simulink model "COMP_POS_CMD"  (R2026b)
settings: Solver=VariableStepAuto
libraries: simulink_extras x1
settings Model: Creator=bhorton  LastModifiedBy=bhorton

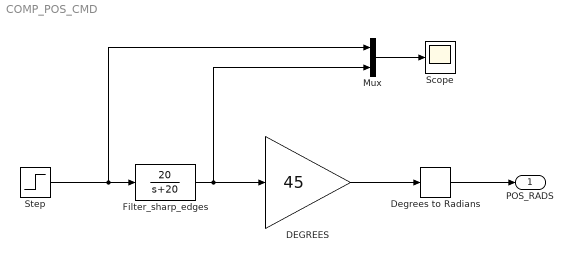
== system COMP_POS_CMD ==
  DEGREES : Gain  Gain=45
  Degrees to Radians : simulink_extras/Transformations/Degrees to Radians
  Filter_sharp_edges : TransferFcn  Numerator=[20]  Denominator=[1 20]
  Mux : Mux  Inputs=2
  Scope : Scope
      settings: ActiveDisplayYMinimum=-0.0343389396209719  ActiveDisplayYMaximum=1.0137019750266969
  Step : Step  Time=5  SampleTime=0
      settings: AttributesFormatString=Step time = %<Time> (secs)
  POS_RADS : Outport
  wires:
  Step/1 -> Mux/1, Filter_sharp_edges/1
  Filter_sharp_edges/1 -> Mux/2, DEGREES/1
  Mux/1 -> Scope/1
  DEGREES/1 -> Degrees to Radians/1
  Degrees to Radians/1 -> POS_RADS/1
